simulink model "detumbling_group24"  (R2023b)
settings: Solver=ode4  StartTime=0.0  StopTime=stopTime  FixedStep=0.1  RelTol=1e-3
values from neighbouring files (symbols this model uses):
  a = 6939    [Air_Drag_script.m]    (also in main.m = 6939.063; main_group24.m = 6939.063)
  A0 = eye(3)    [Air_Drag_script.m]    (also in main_group24.m)
  ARW = 0.15    [main_group24.m]
  by = 0.1    [main_group24.m]
  bz = 0.1    [main_group24.m]
  c = 2.99792*10^8    (= 299792000)    [main.m]    (also in main_group24.m)
  e = 0    [Air_Drag_script.m]    (also in main.m = 0.001304; main_group24.m = 0.001304)
  G = [gn, gm, gvali, gsvi]    [main.m]    (also in main_group24.m)
  GyroSampleRate = 10    [main_group24.m]
  H = [hn, hm, hvali, hsvi]    [main.m]    (also in main_group24.m)
  i = deg2rad(97.5307)    [Air_Drag_script.m]    (also in main.m; main_group24.m)
  inertia1 = Iz-Iy    (= -0.016811111)    [main.m]    (also in main_group24.m = -0.0205003333333)
  inertia2 = Ix-Iz    (= 0.033125546)    [main.m]    (also in main_group24.m = 0.0205003333333)
  inertia3 = Iy-Ix    (= -0.016314435)    [main.m]    (also in main_group24.m = 0)
  Inertia_matrix = [Ix 0 0; 0 Iy 0; 0 0 Iz]    [main.m]
  Inverse_inertia = inv(Inertia_matrix)    [main.m]
  Ix = J(1,1)    [Air_Drag_script.m]    (also in data_mass.m = 0.0755003333333; main.m = 0.057749855; main_group24.m = 0.0755003333333)
  Iy = J(2,2)    [Air_Drag_script.m]    (also in data_mass.m = 0.0755003333333; main.m = 0.04143542; main_group24.m = 0.0755003333333)
  Iz = J(3,3)    [Air_Drag_script.m]    (also in data_mass.m = 0.055; main.m = 0.024624309; main_group24.m = 0.055)
  Ld = 1e-5    (= 1e-05)    [main_group24.m]
  Lw = 0.8    [main_group24.m]
  m = [0.1; 0.1; 0.1]    [main.m]    (also in main_group24.m)
  MB = [4; 0.1; 0.1; 0.3]    [main.m]    (also in main_group24.m)
  MMnoise = 15e-9*[1; 1; 1]    [main_group24.m]
  MMSampleRate = 1    [main_group24.m]
  mu = 3.98600433e+5    (= 398600.433)    [main.m]    (also in main_group24.m)
  n = 0.0011    [Air_Drag_script.m]    (also in main.m = sqrt(mu/a^3); main_group24.m = sqrt(mu/a^3))
  q0 = [ 1 1 1 1 ]'    [Air_Drag_script.m]    (also in main_group24.m = [0 0 0 1]')
  R_e = 6378    [main.m]    (also in main_group24.m)
  rho_d_MB = 0.1    [main.m]    (also in main_group24.m)
  rho_d_SP = 0.1    [main.m]    (also in main_group24.m)
  rho_s_MB = 0.5    [main.m]    (also in main_group24.m)
  rho_s_SP = 0.1    [main.m]    (also in main_group24.m)
  RRW = 0.3    [main_group24.m]
  SP = [1; 0.3; 0.1; 0.01]    [main.m]    (also in main_group24.m = [0.25; 0.1; 0.3; 0.01])
  w0 = [0 0 0]'    [Air_Drag_script.m]    (also in main.m = [wx0; wy0; wz0]; main_group24.m = [wx0; wy0; wz0])
undefined symbols (not defined in the file or in its folder): thrust
libraries: matrix_library x8, vrlib x2, simulink_extras x1, slpidlib x1, sharedutil x1
(part 1 of 3)
settings Model: Creator=hp  LastModifiedBy=hp

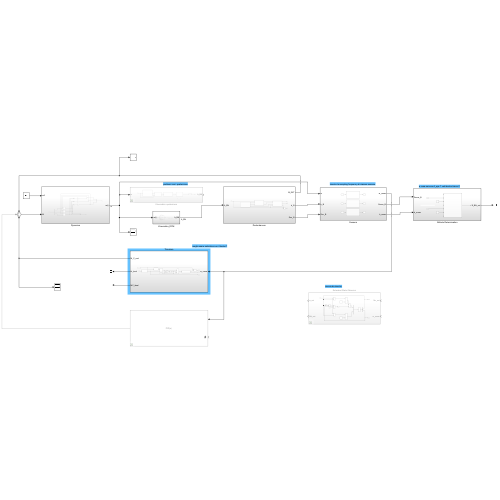
[thumbnail: Simulink's stored preview of the top-level diagram]
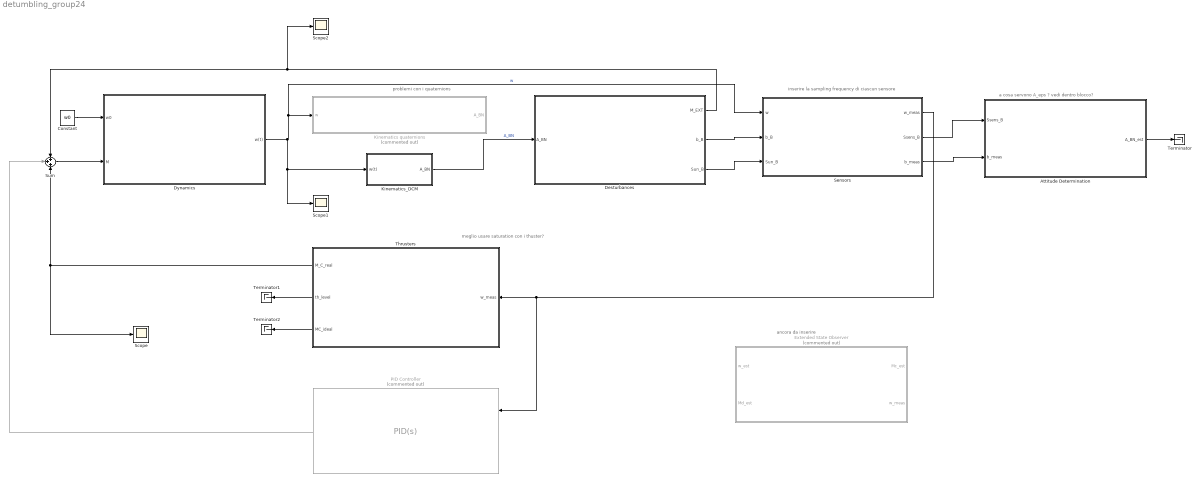
== system detumbling_group24 ==
  note: meglio usare saturation con i thuster?
  note: a cosa servono A_eps ? vedi dentro blocco?
  note: inserire la sampling frequency di ciascun sensore
  note: ancora da inserire
  note: problemi con i quaternions
  Attitude Determination : Subsystem
  Constant : Constant  Value=w0  VectorParams1D=off
  Desturbances : Subsystem
  Dynamics : Subsystem
  Extended State Observer : Subsystem  Commented=on
  Kinematics quaternions : Subsystem  Commented=on
  Kinematics_DCM : Subsystem
  PID Controller : slpidlib/PID Controller  Commented=on  Controller=PID  Form=Parallel  TimeDomain=Continuous-time  UseExternalTs=off  SampleTime=-1  IntegratorMethod=Forward Euler  FilterMethod=Forward Euler  ControllerParametersSource=internal  P=1000  I=0.1  UseKiTs=off  D=20  N=100  UseFilter=on  TunerSelectOption=Transfer Function Based (PID Tuner App)  InitialConditionSource=internal  InitialConditionForIntegrator=0  InitialConditionForFilter=0  DifferentiatorICPrevScaledInput=0  ExternalReset=level  TrackingMode=off  Kt=1  LimitOutput=off  SatLimitsSource=internal  UpperSaturationLimit=inf  LowerSaturationLimit=-inf  LinearizeAsGain=on  AntiWindupMode=none  Kb=1  LimitIntegrator=off  UpperIntegratorSaturationLimit=inf  LowerIntegratorSaturationLimit=-inf  POutMin=[]  POutMax=[]  IOutMin=[]  IOutMax=[]  DOutMin=[]  DOutMax=[]  NOutMin=[]  NOutMax=[]  SumOutMin=[]  SumOutMax=[]  SaturationOutMin=[]  SaturationOutMax=[]  PParamMin=[]  PParamMax=[]  IParamMin=[]  IParamMax=[]  DParamMin=[]  DParamMax=[]  NParamMin=[]  NParamMax=[]  KbParamMin=[]  KbParamMax=[]  KtParamMin=[]  KtParamMax=[]  KbOutMin=[]  KbOutMax=[]  KtOutMin=[]  KtOutMax=[]  IntegratorOutMin=[]  IntegratorOutMax=[]  FilterOutMin=[]  FilterOutMax=[]  SumI1OutMin=[]  SumI1OutMax=[]  SumI2OutMin=[]  SumI2OutMax=[]  SumI3OutMin=[]  SumI3OutMax=[]  SumI4OutMin=[]  SumI4OutMax=[]  SumDOutMin=[]  SumDOutMax=[]  DifferentiatorOutMin=[]  DifferentiatorOutMax=[]  FilterDiffOutCoefMin=[]  FilterDiffOutCoefMax=[]  ReciprocalOutMin=[]  ReciprocalOutMax=[]  SumDenOutMin=[]  SumDenOutMax=[]  SumNumOutMin=[]  SumNumOutMax=[]  DivideOutMin=[]  DivideOutMax=[]  UdiffTsProdOutMin=[]  UdiffTsProdOutMax=[]  NTsProdOutMin=[]  NTsProdOutMax=[]  UintegralTsProdOutMin=[]  UintegralTsProdOutMax=[]  UngainTsProdOutMin=[]  UngainTsProdOutMax=[]  ClampingZeroOutDataTypeStr=Inherit: Inherit via back propagation  ClampingZeroOutMin=[]  ClampingZeroOutMax=[]  FilterDenConstantOutDataTypeStr=Inherit: Inherit via back propagation  FilterDenConstantOutMin=[]  FilterDenConstantOutMax=[]  PCopyOutDataTypeStr=Inherit: Inherit via back propagation  PCopyOutMin=[]  PCopyOutMax=[]  NCopyOutDataTypeStr=Inherit: Inherit via back propagation  NCopyOutMin=[]  NCopyOutMax=[]  IntegratorContinuousStateAttributes=''  IntegratorStateMustResolveToSignalObject=off  IntegratorRTWStateStorageClass=Auto  FilterContinuousStateAttributes=''  FilterStateMustResolveToSignalObject=off  FilterRTWStateStorageClass=Auto  ParallelPVariant=InternalParameters  IdealPVariant=Disabled  IVariant=InternalParameters  DVariant=InternalParameters  IntegratorVariant=Continuous  SatVariant=Disabled  AWVariant=Passthrough  PCopyVariant=Disabled  TRVariant=Disabled  FdbkBlocksVariant=Forward  IdealPFdbkVariant=Disabled  SatFdbkVariant=Disabled  DerivativeFilterVariant=ContFilter  NVariant=InternalParameters  NCopyVariant=Disabled  FilterICVariant=InternalICsFilter  IntegratorICVariant=InternalICs  ExternalResetVariant=ExternalReset  TRSumVariant=Passthrough  SumFdbkVariant=Disabled  SumVariant=Sum_PID  TsampFilterVariant=InternalTs  TsampNgainVariant=Passthrough  TsampIntegralVariant=Disabled_SignalSpec  ExternalSaturationOutDataTypeStr=Inherit: Same as second input
  Scope : Scope
  Scope1 : Scope
  Scope2 : Scope
  Sensors : Subsystem
  Sum : Sum  Inputs=+++
  Terminator : Terminator
  Terminator1 : Terminator
  Terminator2 : Terminator
  Thrusters : Subsystem
  wires:
  Sensors/3(b_meas) -> Attitude Determination/2(b_meas)
  Sensors/2(Ssens_B) -> Attitude Determination/1(Ssens_B)
  Dynamics/1(w(t)) -> Scope1/1, Kinematics_DCM/1(w(t)), Sensors/1(w), Kinematics quaternions/1(w)  "w"
  Desturbances/2(b_B) -> Sensors/2(b_B)
  Sensors/1(w_meas) -> PID Controller/1, Thrusters/1(w_meas)
  Desturbances/3(Sun_B) -> Sensors/3(Sun_B)
  Sum/1 -> Dynamics/2(M)
  Thrusters/1(M_C_real) -> Sum/3, Scope/1
  Desturbances/1(M_EXT) -> Scope2/1, Sum/1
  Attitude Determination/1(A_BN_est) -> Terminator/1
  Thrusters/3(MC_ideal) -> Terminator2/1
  Thrusters/2(th_level) -> Terminator1/1
  Constant/1 -> Dynamics/1(w0)
  Kinematics_DCM/1(A_BN) -> Desturbances/1(A_BN)  "A_BN"
  PID Controller/1 -> Sum/2

== system detumbling_group24/Attitude Determination ==
  note: perchè aggiungere ancora A_eps?????
  Ssens_B : Inport
  b_meas : Inport  Port=2
  Attitude Determination : MATLAB Function  TreatAsAtomicUnit=on
  Constant : Constant
  Constant1 : Constant
  A_BN_est : Outport
  wires:
  Attitude Determination/1(A_BN_est) -> A_BN_est/1  "A_BN_est"
  b_meas/1 -> Attitude Determination/2(b_N)
  Ssens_B/1 -> Attitude Determination/5(r_N)
  Constant1/1 -> Attitude Determination/6(accuracy2)
  Constant/1 -> Attitude Determination/3(accuracy1)

== system detumbling_group24/Desturbances ==
  A_BN : Inport
  External Torques : Subsystem
  MatrixMultiply : Product  Multiplication=Matrix(*)
  Orbital Mechanics : Subsystem
  Relative Attitude : Subsystem
  M_EXT : Outport
  b_B : Outport  Port=2
  Sun_B : Outport  Port=3
  wires:
  Relative Attitude/1(A_BL.) -> External Torques/1(A_BL)
  Relative Attitude/2(r_L) -> External Torques/2(r_L)
  A_BN/1 -> External Torques/4(A_BN), MatrixMultiply/1, Relative Attitude/1(A_BN_ideal)
  Orbital Mechanics/1(theta) -> Relative Attitude/2(theta)
  Orbital Mechanics/2(r_N) -> Relative Attitude/3(r_N)
  Orbital Mechanics/3(r) -> External Torques/3(r)
  External Torques/1(M_EXT) -> M_EXT/1
  External Torques/2(b_B) -> b_B/1
  External Torques/3(Sun_N) -> MatrixMultiply/2
  MatrixMultiply/1 -> Sun_B/1

== system detumbling_group24/Dynamics ==
  w0 : Inport
  M : Inport  Port=2
  Demux : Demux  Outputs=3
  Demux1 : Demux  Outputs=3
  Gain : Gain  Gain=(Iy-Iz)/Ix
  Gain1 : Gain  Gain=(Iz-Ix)/Iy
  Gain2 : Gain  Gain=(Ix-Iy)/Iz
  Sum : Sum  Inputs=|++
  Sum1 : Sum  Inputs=|++
  Sum2 : Sum  Inputs=|++
  Vector Concatenate : Concatenate  NumInputs=3  Mode=Multidimensional array
  XZ : Product
  YX : Product
  ZY : Product
  wx : Integrator  InitialConditionSource=external
  wy : Integrator  InitialConditionSource=external
  wz : Integrator  InitialConditionSource=external
  w(t) : Outport
  wires:
  XZ/1 -> Gain1/1
  Demux/2 -> wy/2  "wy0"
  wx/1 -> XZ/1, Vector Concatenate/1, YX/1
  w0/1 -> Demux/1
  wy/1 -> Vector Concatenate/2, YX/2, ZY/2
  Demux/1 -> wx/2  "wx0"
  wz/1 -> ZY/1, Vector Concatenate/3, XZ/2
  YX/1 -> Gain2/1
  Demux/3 -> wz/2  "wz0"
  ZY/1 -> Gain/1
  Vector Concatenate/1 -> w(t)/1
  Gain2/1 -> Sum2/1
  Gain1/1 -> Sum1/1
  Gain/1 -> Sum/1
  Sum/1 -> wx/1
  Sum1/1 -> wy/1
  Sum2/1 -> wz/1
  Demux1/1 -> Sum/2  "Mx"
  Demux1/2 -> Sum1/2  "My"
  Demux1/3 -> Sum2/2  "Mz"
  M/1 -> Demux1/1

== system detumbling_group24/Extended State Observer ==
  Mc_est : Inport
  w_meas : Inport  Port=2
  Constant4 : Constant  Value=Lw
  Constant5 : Constant  Value=Ld
  Cross Product : vrlib/Utilities/Cross Product
  Demux1 : Demux  Outputs=2
  Gain : Gain  Gain=Inertia_matrix  Multiplication=Matrix(K*u)
  Gain1 : Gain  Gain=Inverse_inertia  Multiplication=Matrix(K*u)
  Integrator : Integrator  InitialCondition=[w0; [0; 0; 0]]
  Mux : Mux  Inputs=2
  Product4 : Product
  Product5 : Product
  Sum4 : Sum  Inputs=+-
  Sum5 : Sum  Inputs=+-
  Sum6 : Sum
  Sum7 : Sum  Inputs=+++
  w_est : Outport
  Md_est : Outport  Port=2
  wires:
  Gain/1 -> Cross Product/1
  Sum5/1 -> Product5/1
  Constant5/1 -> Product5/2
  Cross Product/1 -> Sum7/1
  Product5/1 -> Mux/2
  Demux1/1 -> Sum5/2, Cross Product/2, Gain/1, Sum4/2, w_est/1
  Sum7/1 -> Gain1/1
  Gain1/1 -> Sum6/2
  Product4/1 -> Sum6/1
  Sum6/1 -> Mux/1
  Demux1/2 -> Md_est/1, Sum7/2
  Mux/1 -> Integrator/1
  Mc_est/1 -> Sum7/3
  w_meas/1 -> Sum5/1, Sum4/1
  Integrator/1 -> Demux1/1
  Constant4/1 -> Product4/2
  Sum4/1 -> Product4/1

== system detumbling_group24/Kinematics quaternions ==
  w : Inport
  A_matrix : Subsystem
  Create Omega Matrix : Subsystem
  Kinematics_quaternions : Subsystem
  Normalizer : Subsystem
  Subsystem : Subsystem  Commented=on
  w_at_matrix : Subsystem
  A_BN : Outport
  wires:
  Kinematics_quaternions/1(q_vect) -> A_matrix/1(q_vect)
  A_matrix/1(A_BN) -> Normalizer/1(A_BN)
  w/1 -> Create Omega Matrix/2(w), w_at_matrix/1(w(t))
  Create Omega Matrix/1(Omega) -> Kinematics_quaternions/1(Omega)  "Omega"
  w_at_matrix/1("[-w^]") -> Create Omega Matrix/1("[w^]")  "[-w^]"
  Normalizer/1(Out1) -> A_BN/1

== system detumbling_group24/Kinematics_DCM ==
  w(t) : Inport
  Constant : Constant  Value=0
  Constant1 : Constant  Value=0
  Constant2 : Constant  Value=0
  Demux : Demux  Outputs=3
  Integrator : Integrator  InitialCondition=A0
  Matrix Concatenate : Concatenate  NumInputs=3  Mode=Multidimensional array
  MatrixMultiply : Product  Multiplication=Matrix(*)
  Multiply{,1..3} (4 alike) : Gain  Gain=-1
  Mux : Mux  Inputs=3
  Mux1 : Mux  Inputs=3
  Mux2 : Mux  Inputs=3
  Reshape : Reshape  OutputDimensionality=Row vector (2-D)
  Reshape1 : Reshape  OutputDimensionality=Row vector (2-D)
  Reshape2 : Reshape  OutputDimensionality=Row vector (2-D)
  Scope : Scope
  Subsystem : Subsystem
  A_BN : Outport
  wires:
  w(t)/1 -> Demux/1  "omega"
  MatrixMultiply/1 -> Integrator/1  "dA_dt"
  Matrix Concatenate/1 -> Multiply3/1  "omega_hat"
  Constant/1 -> Mux/1
  Demux/3 -> Mux1/1, Multiply/1  "w_z"
  Multiply/1 -> Mux/2
  Demux/2 -> Mux/3, Multiply2/1  "w_y"
  Constant1/1 -> Mux1/2
  Demux/1 -> Mux2/2, Multiply1/1  "w_x"
  Multiply1/1 -> Mux1/3
  Constant2/1 -> Mux2/3
  Multiply2/1 -> Mux2/1
  Mux/1 -> Reshape/1
  Mux1/1 -> Reshape1/1
  Mux2/1 -> Reshape2/1
  Multiply3/1 -> MatrixMultiply/1
  Reshape/1 -> Matrix Concatenate/1
  Reshape1/1 -> Matrix Concatenate/2
  Reshape2/1 -> Matrix Concatenate/3
  Integrator/1 -> Subsystem/1(In1), MatrixMultiply/2  "A_BN"
  Subsystem/1(Out2) -> Scope/1, A_BN/1

== system detumbling_group24/Sensors ==
  w : Inport
  b_B : Inport  Port=2
  Sun_B : Inport  Port=3
  Gyroscope : Subsystem
  Magnetometer : Subsystem
  Sun Sensor : Subsystem
  w_meas : Outport
  Ssens_B : Outport  Port=2
  b_meas : Outport  Port=3
  wires:
  w/1 -> Gyroscope/1(w)
  Gyroscope/1(w_meas) -> w_meas/1
  Sun Sensor/1(Ssens_B) -> Ssens_B/1
  Sun_B/1 -> Sun Sensor/1(Sun_B)
  b_B/1 -> Magnetometer/1(b_B)
  Magnetometer/1(MM_meas) -> b_meas/1

== system detumbling_group24/Thrusters ==
  w_meas : Inport
  Constant : Constant  Value=thrust.w
  Constant1 : Constant  Value=thrust.R
  Divide : Product  Inputs=*/
  Ideal control (detumbling) : Subsystem
  MATLAB Function : MATLAB Function  TreatAsAtomicUnit=on
  MATLAB Function1 : MATLAB Function  TreatAsAtomicUnit=on
  Matrix Multiply : Product  Multiplication=Matrix(*)
  Matrix Multiply1 : Product  Multiplication=Matrix(*)
  Max of Elements : MinMax  Function=max
  Product : Product
  Sum : Sum
  M_C_real : Outport
  th_level : Outport  Port=2
  MC_ideal : Outport  Port=3
  wires:
  Constant/1 -> Divide/2, Product/2  "w"
  Product/1 -> Sum/2
  Divide/1 -> Max of Elements/1
  Max of Elements/1 -> Product/1  "gamma"
  Ideal control (detumbling)/1(MC_ideal) -> MC_ideal/1, Matrix Multiply/2
  MATLAB Function1/1(y) -> Matrix Multiply/1
  Matrix Multiply1/1 -> M_C_real/1
  Sum/1 -> MATLAB Function/1(u_c)  "deal"
  Matrix Multiply/1 -> Divide/1, Sum/1
  MATLAB Function/1(u_c_real) -> Matrix Multiply1/2  "real"
  MATLAB Function/2(th_level) -> th_level/1
  w_meas/1 -> Ideal control (detumbling)/1(w)
  Constant1/1 -> Matrix Multiply1/1, MATLAB Function1/1(u)

== system detumbling_group24/Desturbances/External Torques ==
  A_BL : Inport
  r_L : Inport  Port=2
  r : Inport  Port=3
  A_BN : Inport  Port=4
  Constant : Constant  Value=MB
  Constant1 : Constant  Value=SP
  M_GG : Subsystem
  Magnetic field : Subsystem
  Solar radiation : Subsystem
  Sum of Elements : Sum  Inputs=+++
  To Workspace : ToWorkspace  VariableName=M_GG  SaveFormat=Timeseries  SampleTime=-1
  To Workspace1 : ToWorkspace  VariableName=M_SRP  SaveFormat=Timeseries  SampleTime=-1
  To Workspace2 : ToWorkspace  VariableName=M_MAG  SaveFormat=Timeseries  SampleTime=-1
  M_EXT : Outport
  b_B : Outport  Port=2
  Sun_N : Outport  Port=3
  wires:
  r/1 -> M_GG/2(r)
  Constant/1 -> Solar radiation/2(MB)
  Constant1/1 -> Solar radiation/3(SP)
  A_BN/1 -> Solar radiation/1(A_BN), Magnetic field/2(A_BN)
  Magnetic field/1(M_MAG) -> To Workspace2/1, Sum of Elements/3
  Sum of Elements/1 -> M_EXT/1
  A_BL/1 -> M_GG/1(A_BL)
  r_L/1 -> Magnetic field/1(r_L)
  M_GG/1(M_GG1) -> Sum of Elements/1, To Workspace/1
  Solar radiation/1(T_SRP) -> To Workspace1/1, Sum of Elements/2
  Magnetic field/2(b_B) -> b_B/1
  Solar radiation/2(Sun_N) -> Sun_N/1

== system detumbling_group24/Desturbances/Orbital Mechanics ==
  Sat Position magnitude : Subsystem
  Sat True Anomaly : Subsystem
  Sat position vector in inertial frame : Subsystem
  theta : Outport
  r_N : Outport  Port=2
  r : Outport  Port=3
  wires:
  Sat True Anomaly/1(theta) -> Sat position vector in inertial frame/2(theta), theta/1, Sat Position magnitude/1(theta)  "theta"
  Sat Position magnitude/1(r) -> r/1, Sat position vector in inertial frame/1(r)
  Sat position vector in inertial frame/1(r_N) -> r_N/1  "r_N"

== system detumbling_group24/Desturbances/Relative Attitude ==
  A_BN_ideal : Inport
  theta : Inport  Port=2
  r_N : Inport  Port=3
  A_BL : Subsystem
  A_LN : Subsystem
  MatrixMultiply : Product  Multiplication=Matrix(*)
  A_BL. : Outport
  r_L : Outport  Port=2
  wires:
  A_LN/1(A_LN) -> MatrixMultiply/1, A_BL/2(A_LN)
  theta/1 -> A_LN/1(theta)
  A_BN_ideal/1 -> A_BL/1(A_BN)
  A_BL/1(A_BL) -> A_BL./1
  r_N/1 -> MatrixMultiply/2
  MatrixMultiply/1 -> r_L/1

== system detumbling_group24/Kinematics quaternions/A_matrix ==
  q_vect : Inport
  Add : Sum  Inputs=++-
  Constant : Constant  Value=0
  Constant1 : Constant  Value=0
  Constant2 : Constant  Value=0
  Demux : Demux
  I : Constant  Value=eye(3)
  Matrix Concatenate : Concatenate  NumInputs=3  Mode=Multidimensional array
  MatrixMultiply : Product  Multiplication=Matrix(*)
  MatrixMultiply1 : Product
  MatrixMultiply2 : Product  Multiplication=Matrix(*)
  MatrixMultiply3 : Product
  Multiply : Gain  Gain=-1
  Multiply1 : Gain  Gain=-1
  Multiply2 : Gain  Gain=-1
  Multiply3 : Gain  Gain=2
  Multiply4 : Gain  Gain=2
  Mux{,1..3} (4 alike) : Mux  Inputs=3
  Reshape : Reshape  OutputDimensionality=Row vector (2-D)
  Reshape1 : Reshape  OutputDimensionality=Row vector (2-D)
  Reshape2 : Reshape  OutputDimensionality=Row vector (2-D)
  Square : Math  Operator=square
  Subtract : Sum  Inputs=-+
  Transpose : Math  Operator=transpose
  A_BN : Outport
  wires:
  q_vect/1 -> Demux/1
  Demux/1 -> Mux3/1, Mux2/2, Multiply1/1  "q1"
  Demux/2 -> Mux3/2, Mux/3, Multiply2/1  "q2"
  Demux/3 -> Mux3/3, Multiply/1, Mux1/1  "q3"
  Demux/4 -> Square/1, Multiply4/1  "q4"
  Mux/1 -> Reshape/1
  Reshape/1 -> Matrix Concatenate/1
  Mux1/1 -> Reshape1/1
  Mux2/1 -> Reshape2/1
  Reshape1/1 -> Matrix Concatenate/2
  Reshape2/1 -> Matrix Concatenate/3
  Multiply/1 -> Mux/2
  Constant1/1 -> Mux1/2
  Multiply1/1 -> Mux1/3
  Multiply2/1 -> Mux2/1
  Constant2/1 -> Mux2/3
  Matrix Concatenate/1 -> MatrixMultiply3/2  "q_hat"
  Mux3/1 -> MatrixMultiply2/1, Transpose/1, MatrixMultiply/2  "q_bar"
  Transpose/1 -> MatrixMultiply2/2, MatrixMultiply/1
  Square/1 -> Subtract/2
  MatrixMultiply/1 -> Subtract/1
  Subtract/1 -> MatrixMultiply1/1
  I/1 -> MatrixMultiply1/2
  MatrixMultiply2/1 -> Multiply3/1
  Multiply4/1 -> MatrixMultiply3/1
  Multiply3/1 -> Add/1
  MatrixMultiply1/1 -> Add/2
  MatrixMultiply3/1 -> Add/3
  Add/1 -> A_BN/1
  Constant/1 -> Mux/1

== system detumbling_group24/Kinematics quaternions/Create Omega Matrix ==
  "[w^]" : Inport
  w : Inport  Port=2
  " Col added" : Concatenate  Mode=Multidimensional array  ConcatenateDimension=2
  " Row added" : Concatenate  Mode=Multidimensional array
  Constant : Constant  Value=0
  Gain : Gain  Gain=-1
  Transpose : Math  Operator=transpose
  Vector Concatenate : Concatenate
  Omega : Outport
  wires:
  w/1 -> Transpose/1, Vector Concatenate/1
  Constant/1 -> Vector Concatenate/2
  Transpose/1 -> Gain/1
  "[w^]"/1 -> " Row added"/1
  " Row added"/1 -> " Col added"/1
  Vector Concatenate/1 -> " Col added"/2
  Gain/1 -> " Row added"/2
  " Col added"/1 -> Omega/1

== system detumbling_group24/Kinematics quaternions/Kinematics_quaternions ==
  Omega : Inport
  Constant : Constant  Value=q0  VectorParams1D=off
  Gain : Gain  Gain=0.5
  Integrator : Integrator  InitialConditionSource=external  InitialCondition=q0
  Omega*q(t) : Product  Multiplication=Matrix(*)
  Scope : Scope
  q_vect : Outport
  wires:
  Gain/1 -> Scope/1, q_vect/1, Integrator/1
  Integrator/1 -> Omega*q(t)/2  "q(t)"
  Omega*q(t)/1 -> Gain/1
  Omega/1 -> Omega*q(t)/1
  Constant/1 -> Integrator/2

== system detumbling_group24/Kinematics quaternions/Normalizer ==
  A_BN : Inport
  Gain : Gain  Gain=1.5
  Gain1 : Gain  Gain=0.5
  MatrixMultiply : Product  Multiplication=Matrix(*)
  MatrixMultiply1 : Product  Multiplication=Matrix(*)
  Sum : Sum  Inputs=+-
  Transpose : matrix_library/Transpose
  Out1 : Outport
  wires:
  A_BN/1 -> Transpose/1, MatrixMultiply/1, Gain/1, MatrixMultiply1/2
  Gain/1 -> Sum/1
  Sum/1 -> Out1/1
  Transpose/1 -> MatrixMultiply/2
  MatrixMultiply/1 -> MatrixMultiply1/1
  MatrixMultiply1/1 -> Gain1/1
  Gain1/1 -> Sum/2

== system detumbling_group24/Kinematics quaternions/Subsystem ==
  q_vect : Inport
  Demux : Demux
  From{,1..5} (6 alike) : From
  Goto{,1..8} (9 alike) : Goto
  Square{,1..3} (4 alike) : Math  Operator=square
  q1 q2 : Product
  q1 q3 : Product
  q1 q4 : Product
  q2 q4 : Product
  q3 q4 : Product
  Out1 : Outport
  wires:
  q_vect/1 -> Demux/1
  Demux/1 -> q1 q4/1, Square/1, q1 q3/1, q1 q2/1  "q1"
  Demux/2 -> Square1/1, q1 q2/2  "q2"
  Demux/3 -> q3 q4/2, Square2/1, q1 q3/2  "q3"
  Demux/4 -> q1 q4/2, q3 q4/1, Square3/1  "q4"
  q1 q2/1 -> Goto/1
  q1 q3/1 -> Goto1/1
  Square/1 -> Goto2/1
  Square1/1 -> Goto3/1
  Square2/1 -> Goto4/1
  Square3/1 -> Goto5/1
  q3 q4/1 -> Goto6/1
  q2 q4/1 -> Goto7/1
  q1 q4/1 -> Goto8/1

== system detumbling_group24/Kinematics quaternions/w_at_matrix ==
  w(t) : Inport
  Constant : Constant  Value=0  VectorParams1D=off
  Constant1 : Constant  Value=0
  Constant2 : Constant  Value=0
  Demux : Demux  Outputs=3
  Gain3 : Gain  Gain=-1
  Gain4 : Gain  Gain=-1
  Gain5 : Gain  Gain=-1
  Matrix Concatenate1 : Concatenate  NumInputs=3  Mode=Multidimensional array  ConcatenateDimension=2
  Mux1 : Mux  Inputs=3
  Mux2 : Mux  Inputs=3
  Mux3 : Mux  Inputs=3
  "[-w^]" : Outport
  wires:
  Demux/2 -> Mux1/3, Gain5/1  "wy"
  Gain3/1 -> Mux1/2
  Matrix Concatenate1/1 -> "[-w^]"/1
  Constant2/1 -> Mux3/3
  Demux/3 -> Mux2/1, Gain3/1  "wz"
  Constant1/1 -> Mux2/2
  Demux/1 -> Gain4/1, Mux3/2  "wx"
  Gain4/1 -> Mux2/3
  Mux1/1 -> Matrix Concatenate1/1
  Mux2/1 -> Matrix Concatenate1/2
  Gain5/1 -> Mux3/1
  Constant/1 -> Mux1/1
  Mux3/1 -> Matrix Concatenate1/3
  w(t)/1 -> Demux/1

== system detumbling_group24/Kinematics_DCM/Subsystem ==
  In1 : Inport
  Matrix Multiply : Product  Multiplication=Matrix(*)
  Matrix Multiply1 : Product  Multiplication=Matrix(*)
  Multiply : Gain  Gain=3/2
  Multiply1 : Gain  Gain=1/2
  Subtract : Sum  Inputs=+-
  Transpose : Math  Operator=transpose
  Out2 : Outport
  wires:
  Subtract/1 -> Out2/1
  Multiply1/1 -> Subtract/2
  Matrix Multiply1/1 -> Multiply1/1
  Multiply/1 -> Subtract/1
  Transpose/1 -> Matrix Multiply/2
  Matrix Multiply/1 -> Matrix Multiply1/1
  In1/1 -> Matrix Multiply1/2, Matrix Multiply/1, Multiply/1, Transpose/1  "A"

== system detumbling_group24/Sensors/Gyroscope ==
  note: w_BN_measured = G(w_B) A_eps w_BN + n + b
  w : Inport
  ARW : RandomNumber  Variance=(deg2rad(ARW)/sqrt(3600)/sqrt(1/GyroSampleRate))^2*[1;1;1]  SampleTime=1/GyroSampleRate
  Integrator : Integrator
  RRW : RandomNumber  Variance=(deg2rad(RRW)/3600/sqrt(1/GyroSampleRate))^2* [1;1;1]  SampleTime=1/GyroSampleRate
  Sum : Sum  Inputs=+++
  w_meas : Outport
  wires:
  RRW/1 -> Integrator/1  "b_dot"
  ARW/1 -> Sum/2  "n"
  Integrator/1 -> Sum/3  "b"
  Sum/1 -> w_meas/1
  w/1 -> Sum/1

== system detumbling_group24/Sensors/Magnetometer ==
  b_B : Inport
  Constant : Constant  Value=MMnoise
  MatrixMultiply : Product  Multiplication=Matrix(*)
  Subsystem : Subsystem
  Sum : Sum
  MM_meas : Outport
  wires:
  Constant/1 -> Sum/2
  b_B/1 -> Sum/1  "b_B"
  Subsystem/1(A_epsMM) -> MatrixMultiply/1
  Sum/1 -> MatrixMultiply/2
  MatrixMultiply/1 -> MM_meas/1

== system detumbling_group24/Sensors/Sun Sensor ==
  Sun_B : Inport
  Matrix Multiply1 : Product  Multiplication=Matrix(*)
  Subsystem : Subsystem
  Ssens_B : Outport
  wires:
  Sun_B/1 -> Matrix Multiply1/2
  Subsystem/1(A_eps) -> Matrix Multiply1/1  "A_eps"
  Matrix Multiply1/1 -> Ssens_B/1

== system detumbling_group24/Thrusters/Ideal control (detumbling) ==
  w : Inport
  Bracci thrusters : Constant  Value=[bz ; bz ; by]  VectorParams1D=off
  Gain3 : Gain  Gain=-1
  Matrix Multiply : Product
  Product2 : Product
  Sign : Signum
  variable T : MATLAB Function  TreatAsAtomicUnit=on
  MC_ideal : Outport
  wires:
  w/1 -> Sign/1, variable T/1(w)
  Matrix Multiply/1 -> Product2/1
  Product2/1 -> Gain3/1
  variable T/1(T) -> Matrix Multiply/2
  Bracci thrusters/1 -> Matrix Multiply/1
  Sign/1 -> Product2/2
  Gain3/1 -> MC_ideal/1

== system detumbling_group24/Desturbances/External Torques/M_GG ==
  A_BL : Inport
  r : Inport  Port=2
  GG Torque1 : Subsystem
  "c1, c2, c3" : Subsystem
  M_GG1 : Outport
  wires:
  "c1, c2, c3"/1(c1) -> GG Torque1/1(c1)
  "c1, c2, c3"/2(c2) -> GG Torque1/2(c2)
  "c1, c2, c3"/3(c3) -> GG Torque1/3(c3)
  A_BL/1 -> "c1, c2, c3"/1(A_BL)
  GG Torque1/1(M_GG) -> M_GG1/1
  r/1 -> GG Torque1/4(r)

== system detumbling_group24/Desturbances/External Torques/Magnetic field ==
  r_L : Inport
  A_BN : Inport  Port=2
  Clock : Clock
  Constant : Constant  Value=m
  Constant1 : Constant  Value=R_e*1000
  Constant3 : Constant  Value=G
  Constant4 : Constant  Value=H
  Cross Product1 : matrix_library/Cross Product
  MATLAB Function : MATLAB Function  TreatAsAtomicUnit=on
  MatrixMultiply : Product  Multiplication=Matrix(*)
  Reshape1 : Reshape  OutputDimensionality=Column vector (2-D)
  M_MAG : Outport
  b_B : Outport  Port=2
  wires:
  Constant1/1 -> MATLAB Function/2(r)
  Clock/1 -> MATLAB Function/3(t)
  Constant3/1 -> MATLAB Function/4(G)
  MATLAB Function/1(b_N) -> Reshape1/1
  r_L/1 -> MATLAB Function/1(r_LVLH)
  Reshape1/1 -> MatrixMultiply/2
  Constant4/1 -> MATLAB Function/5(H)
  A_BN/1 -> MatrixMultiply/1
  Constant/1 -> Cross Product1/1
  MatrixMultiply/1 -> b_B/1, Cross Product1/2
  Cross Product1/1 -> M_MAG/1

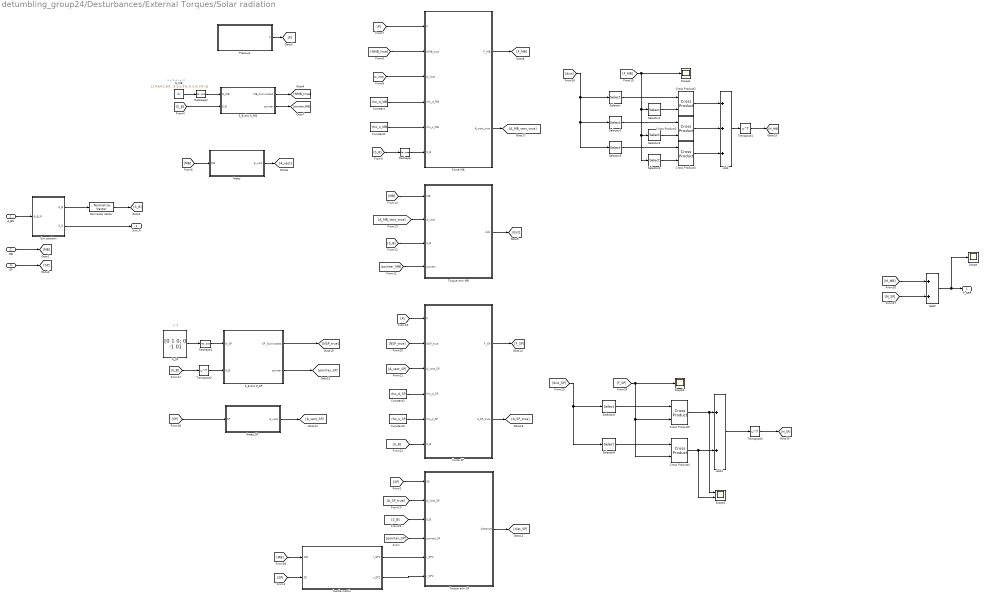
== system detumbling_group24/Desturbances/External Torques/Solar radiation ==
  note: x,y,z,-x,-y,-z
  note: y,-y
  A_BN : Inport
  MB : Inport  Port=2
  SP : Inport  Port=3
  Add : Sum  Inputs=3
  Add1 : Sum
  Add2 : Sum
  Areas : Subsystem
  Areas_SP : Subsystem
  Constant : Constant  Value=rho_d_MB
  Constant1 : Constant  Value=rho_s_MB
  Constant2 : Constant  Value=rho_d_SP
  Constant3 : Constant  Value=rho_s_SP
  Cross Product{1..5} (5 alike) : matrix_library/Cross Product
  Force MB : Subsystem
  Force SP : Subsystem
  Inertia matrix : Subsystem
  N_MB : Constant  Value=[1 0 0;0 1 0;0 0 1;-1 0 0; 0 -1 0; 0 0 -1]  VectorParams1D=off
  N_SP : Constant  Value=[0 1 0; 0 -1 0]  VectorParams1D=off
  Normalize Vector : vrlib/Utilities/Normalize Vector  maxzero=0
  Pressure : Subsystem
  Reshape : Reshape  OutputDimensionality=Column vector (2-D)
  Reshape1 : Reshape  OutputDimensionality=Customize  OutputDimensions=[2,3]
  Reshape2 : Reshape  OutputDimensionality=Customize  OutputDimensions=[6,3]
  S_B dot N_MB : Subsystem
  S_B dot N_SP : Subsystem
  Scope : Scope
  Scope1 : Scope
  Scope2 : Scope  NumInputPorts=2
  Scope3 : Scope
  Selector : Selector  NumberOfDimensions=2  InputPortWidth=3  IndexOptions=Index vector (dialog),Index vector (dialog)  Indices=1,[1 2 3]  OutputSizes=1,1
  Selector1 : Selector  NumberOfDimensions=2  InputPortWidth=3  IndexOptions=Index vector (dialog),Index vector (dialog)  Indices=1,[1 2 3]  OutputSizes=1,1
  Selector2 : Selector  NumberOfDimensions=2  InputPortWidth=3  IndexOptions=Index vector (dialog),Index vector (dialog)  Indices=2,[1 2 3]  OutputSizes=1,1
  Selector3 : Selector  NumberOfDimensions=2  InputPortWidth=3  IndexOptions=Index vector (dialog),Index vector (dialog)  Indices=2,[1 2 3]  OutputSizes=1,1
  Selector4 : Selector  NumberOfDimensions=2  InputPortWidth=3  IndexOptions=Index vector (dialog),Index vector (dialog)  Indices=3,[1 2 3]  OutputSizes=1,1
  Selector5 : Selector  NumberOfDimensions=2  InputPortWidth=3  IndexOptions=Index vector (dialog),Index vector (dialog)  Indices=3,[1 2 3]  OutputSizes=1,1
  Selector6 : Selector  NumberOfDimensions=2  InputPortWidth=3  IndexOptions=Index vector (dialog),Index vector (dialog)  Indices=1,[1 2 3]  OutputSizes=1,1
  Selector8 : Selector  NumberOfDimensions=2  InputPortWidth=3  IndexOptions=Index vector (dialog),Index vector (dialog)  Indices=2,[1 2 3]  OutputSizes=1,1
  Sun position : Subsystem
  Torque arm MB : Subsystem
  Torque arm SP : Subsystem
  Transpose1 : Math  Operator=transpose
  Transpose2 : Math  Operator=transpose
  Transpose3 : Math  Operator=transpose
  T_SRP : Outport
  Sun_N : Outport  Port=2
  wires:
  Sun position/1(S_B) -> Normalize Vector/1
  MB/1 -> [MB]
  N_MB/1 -> Reshape2/1
  [NMB_true] -> Force MB/2(NMB_true)
  S_B dot N_MB/1(MB_illuminated) -> [NMB_true]
  [MB] -> Areas/1(MB)
  [S_B] -> S_B dot N_MB/2(S_B)
  Sun position/2(S_N) -> Sun_N/1
  [P] -> Force MB/1(P)
  Areas/1(A_vect) -> [A_vect]
  Transpose1/1 -> [M_MB]
  Areas_SP/1(A_vect) -> [A_vect_SP]
  Reshape1/1 -> S_B dot N_SP/1(N_SP)
  Transpose3/1 -> [M_SP]
  Selector2/1 -> Cross Product1/1
  [MB] -> Torque arm MB/1(MB)
  Constant3/1 -> Force SP/5(rho_s_SP)
  [F_SP] -> Cross Product5/2, Cross Product4/2, Scope3/1
  [M_MB] -> Add2/1
  [dist_SP] -> Selector6/1, Selector8/1
  [pointer_SP] -> Torque arm SP/4(pointer_SP)
  Cross Product4/1 -> Scope2/2, Add1/2
  [F_MB] -> Scope1/1, Selector4/1, Selector3/1, Selector1/1
  A_BN/1 -> Sun position/1(A_B_N)
  Add1/1 -> Transpose3/1
  Transpose2/1 -> S_B dot N_SP/2(S_B)
  [SP] -> Areas_SP/1(SP)
  [A_SP_true] -> Torque arm SP/2(A_vect_SP)
  Add/1 -> Transpose1/1
  Torque arm SP/1(distance) -> [dist_SP]
  Reshape2/1 -> S_B dot N_MB/1(N_MB)
  Torque arm MB/1(dist) -> [dist]
  S_B dot N_SP/2(pointer) -> [pointer_SP]
  Force MB/1(F_MB) -> [F_MB]
  Selector/1 -> Cross Product2/1
  [S_B] -> Reshape/1
  [P] -> Force SP/1(P)
  [A_vect] -> Force MB/3(A_vect)
  Selector1/1 -> Cross Product2/2
  Constant1/1 -> Force MB/5(rho_s_MB)
  [A_MB_vect_true] -> Torque arm MB/2(A_vect)
  Pressure/1(P) -> [P]
  Normalize Vector/1 -> [S_B]
  Constant2/1 -> Force SP/4(rho_d_SP)
  Constant/1 -> Force MB/4(rho_d_MB)
  Selector8/1 -> Cross Product4/1
  [dist] -> Selector2/1, Selector5/1, Selector/1
  [NSP_true] -> Force SP/2(NSP_true)
  N_SP/1 -> Reshape1/1
  [S_B] -> Torque arm MB/3(S_B)
  Force SP/2(A_SP_true) -> [A_SP_true]
  [S_B] -> Torque arm SP/3(S_B)
  SP/1 -> [SP]
  Selector4/1 -> Cross Product3/2
  S_B dot N_MB/2(pointer) -> [pointer_MB]
  Force MB/2(A_vect_true) -> [A_MB_vect_true]
  [pointer_MB] -> Torque arm MB/4(pointer)
  Add2/1 -> Scope/1, T_SRP/1
  Selector3/1 -> Cross Product1/2
  [S_B] -> Force SP/6(S_B)
  [S_B] -> Transpose2/1
  Cross Product5/1 -> Scope2/1, Add1/1
  [A_vect_SP] -> Force SP/3(A_vect_SP)
  Reshape/1 -> Force MB/6(S_B)
  Cross Product2/1 -> Add/1
  Force SP/1(F_SP) -> [F_SP]
  S_B dot N_SP/1(SP_illuminated) -> [NSP_true]
  Selector6/1 -> Cross Product5/1
  Selector5/1 -> Cross Product3/1
  Cross Product1/1 -> Add/2
  [M_SP] -> Add2/2
  [SP] -> Torque arm SP/1(SP)
  Cross Product3/1 -> Add/3
  [SP] -> Inertia matrix/2(SP)
  [MB] -> Inertia matrix/1(MB)
  Inertia matrix/1(r_SP1) -> Torque arm SP/5(r_SP1)
  Inertia matrix/2(r_SP2) -> Torque arm SP/6(r_SP2)

== system detumbling_group24/Desturbances/Orbital Mechanics/Sat Position magnitude ==
  note: 1+e cos(theta)
  note: a(1-e^2)
  note: Denominator
  note: Numerator
  theta : Inport
  Constant : Constant  Value=a
  Constant1 : Constant
  Constant3 : Constant  Value=e
  Constant4 : Constant
  Constant5 : Constant  Value=e
  Cos : Trigonometry  Operator=cos
  Divide : Product  Inputs=*/
  Product : Product
  Product1 : Product
  Square1 : Math  Operator=square
  Sum : Sum
  Sum1 : Sum  Inputs=+-
  r : Outport
  wires:
  Product1/1 -> Sum/1
  Sum1/1 -> Product/2
  Constant1/1 -> Sum1/1
  Sum/1 -> Divide/2
  Square1/1 -> Sum1/2
  Constant3/1 -> Product1/2
  Constant4/1 -> Sum/2
  Constant/1 -> Product/1
  Constant5/1 -> Square1/1
  Cos/1 -> Product1/1
  Product/1 -> Divide/1
  theta/1 -> Cos/1
  Divide/1 -> r/1

== system detumbling_group24/Desturbances/Orbital Mechanics/Sat True Anomaly ==
  note: (1-e^2)^3/2
  note: n ( 1+e cos(theta))^2
  note: Denominator
  note: Numerator
  Constant : Constant  Value=n
  Constant1 : Constant
  Constant2 : Constant  Value=e
  Constant3 : Constant
  Constant4 : Constant  Value=e
  Constant5 : Constant  Value=3/2
  Cos : Trigonometry  Operator=cos
  Divide : Product  Inputs=*/
  Integrator : Integrator
  Power : Math  Operator=pow
  Product : Product
  Product1 : Product
  Square : Math  Operator=square
  Square1 : Math  Operator=square
  Sum : Sum
  Sum1 : Sum  Inputs=|+-
  theta : Outport
  wires:
  Sum/1 -> Square/1
  Integrator/1 -> theta/1, Cos/1  "theta"
  Square/1 -> Product1/2
  Constant5/1 -> Power/2
  Constant3/1 -> Sum1/1
  Product1/1 -> Divide/1
  Constant/1 -> Product1/1
  Divide/1 -> Integrator/1  "theta_dot"
  Square1/1 -> Sum1/2
  Product/1 -> Sum/2
  Power/1 -> Divide/2
  Constant1/1 -> Sum/1
  Constant2/1 -> Product/1
  Constant4/1 -> Square1/1
  Cos/1 -> Product/2
  Sum1/1 -> Power/1

== system detumbling_group24/Desturbances/Orbital Mechanics/Sat position vector in inertial frame ==
  note: r_N = r [cos(theta)
      | 		sin(theta)cos(i)
      | 		sin(theta)sin(i)]
  r : Inport
  theta : Inport  Port=2
  Cos : Trigonometry  Operator=cos
  Cos1 : Trigonometry  Operator=cos
  Orbit Inclination : Constant  Value=i
  Product : Product
  Product1 : Product
  Product2 : Product
  Sin : Trigonometry
  Sin1 : Trigonometry
  Vector Concatenate : Concatenate  NumInputs=3  Mode=Multidimensional array
  r_N : Outport
  wires:
  Sin/1 -> Product1/1, Product/1
  Product/1 -> Vector Concatenate/2
  Sin1/1 -> Product1/2
  r/1 -> Product2/1
  Orbit Inclination/1 -> Sin1/1, Cos1/1
  Vector Concatenate/1 -> Product2/2
  theta/1 -> Cos/1, Sin/1
  Cos/1 -> Vector Concatenate/1
  Cos1/1 -> Product/2
  Product1/1 -> Vector Concatenate/3
  Product2/1 -> r_N/1

== system detumbling_group24/Desturbances/Relative Attitude/A_BL ==
  A_BN : Inport
  A_LN : Inport  Port=2
  Matrix Multiply : Product  Multiplication=Matrix(*)
  To Workspace : ToWorkspace  VariableName=A_BL  SampleTime=-1
  Transpose1 : matrix_library/Transpose
  A_BL : Outport
  wires:
  A_BN/1 -> Matrix Multiply/1
  A_LN/1 -> Transpose1/1
  Transpose1/1 -> Matrix Multiply/2
  Matrix Multiply/1 -> A_BL/1, To Workspace/1

== system detumbling_group24/Desturbances/Relative Attitude/A_LN ==
  theta : Inport
  Constant : Constant  Value=0
  Constant1 : Constant  Value=[0; 0; 1]
  Constant2 : Constant  Value=[1 0 0; 0 cos(i) sin(i); 0 -sin(i) cos(i)]
  Cos : Trigonometry  Operator=cos
  Gain : Gain  Gain=[1; -1; 1]
  Matrix Concatenate : Concatenate  NumInputs=3  Mode=Multidimensional array  ConcatenateDimension=2
  Product : Product  Multiplication=Matrix(*)
  Selector : Selector  InputPortWidth=3  IndexOptions=Index vector (dialog)  Indices=[3 2 1]  OutputSizes=1
  Selector1 : Selector  InputPortWidth=3  IndexOptions=Index vector (dialog)  Indices=[2 3 1]  OutputSizes=1
  Sin : Trigonometry
  To Workspace : ToWorkspace  VariableName=A_LN  SampleTime=-1
  Vector Concatenate : Concatenate  NumInputs=3
  A_LN : Outport
  wires:
  Matrix Concatenate/1 -> Product/1
  theta/1 -> Sin/1, Cos/1
  Gain/1 -> Matrix Concatenate/1
  Vector Concatenate/1 -> Selector1/1, Selector/1
  Sin/1 -> Vector Concatenate/3
  Selector/1 -> Matrix Concatenate/2
  Selector1/1 -> Gain/1
  Product/1 -> A_LN/1, To Workspace/1
  Constant1/1 -> Matrix Concatenate/3
  Cos/1 -> Vector Concatenate/2
  Constant/1 -> Vector Concatenate/1
  Constant2/1 -> Product/2

== system detumbling_group24/Sensors/Magnetometer/Subsystem ==
  Constant : Constant
  Display : Display
  Gain : Gain  Gain=[1; -1; 1]
  Gain1 : Gain  Gain=[1; 1; -1]
  Gain2 : Gain  Gain=[-1; 1; 1]
  Matrix Concatenate : Concatenate  NumInputs=3  Mode=Multidimensional array  ConcatenateDimension=2
  Random Number : RandomNumber  Variance=deg2rad(0.1)^2  Seed=5  SampleTime=1/MMSampleRate
  Random Number1 : RandomNumber  Variance=deg2rad(0.1)^2  Seed=6  SampleTime=1/MMSampleRate
  Random Number2 : RandomNumber  Variance=deg2rad(0.1)^2  Seed=7  SampleTime=1/MMSampleRate
  Selector : Selector  InputPortWidth=4  IndexOptions=Index vector (dialog)  Indices=[1 4 3]  OutputSizes=1
  Selector1 : Selector  InputPortWidth=4  IndexOptions=Index vector (dialog)  Indices=[4 1 2]  OutputSizes=1
  Selector2 : Selector  InputPortWidth=4  IndexOptions=Index vector (dialog)  Indices=[3 2 1]  OutputSizes=1
  Vector Concatenate : Concatenate  NumInputs=4
  A_epsMM : Outport
  wires:
  Selector2/1 -> Gain2/1
  Selector/1 -> Gain/1
  Gain/1 -> Matrix Concatenate/1
  Random Number/1 -> Vector Concatenate/2
  Matrix Concatenate/1 -> Display/1, A_epsMM/1
  Selector1/1 -> Gain1/1
  Vector Concatenate/1 -> Selector2/1, Selector/1, Selector1/1
  Gain2/1 -> Matrix Concatenate/3
  Constant/1 -> Vector Concatenate/1
  Gain1/1 -> Matrix Concatenate/2
  Random Number2/1 -> Vector Concatenate/4
  Random Number1/1 -> Vector Concatenate/3

== system detumbling_group24/Sensors/Sun Sensor/Subsystem ==
  note: A31
  note: A33
  note: A32
  note: A23
  note: A22
  note: A21
  note: A13
  note: A12
  note: A11
  Cos : Trigonometry  Operator=cos
  Cos1 : Trigonometry  Operator=cos
  Cos2 : Trigonometry  Operator=cos
  Create 3x3 Matrix : sharedutil/Create 3x3 Matrix  aMode=aMode
  Gain1 : Gain  Gain=-1
  Gain3 : Gain  Gain=-1
  Gain4 : Gain
  Product{,1,3,5..6,8,10..11} (8 alike) : Product
  Product{2,4,7,9} (4 alike) : Product  Inputs=3
  Sin : Trigonometry
  Sin1 : Trigonometry
  Sin2 : Trigonometry
  Sum : Sum
  Sum1 : Sum  Inputs=-+
  Sum2 : Sum  Inputs=-+
  Sum3 : Sum
  phi : RandomNumber  Variance=(1/8*pi/180)^2  Seed=2  SampleTime=0.2
  psi : RandomNumber  Variance=(1/8*pi/180)^2  SampleTime=0.2
  th : RandomNumber  Variance=(1/8*pi/180)^2  Seed=1  SampleTime=0.2
  A_eps : Outport
  wires:
  psi/1 -> Cos/1, Sin/1
  th/1 -> Sin1/1, Cos1/1
  phi/1 -> Sin2/1, Cos2/1
  Product2/1 -> Sum/1
  Product1/1 -> Sum/2
  Product3/1 -> Sum1/2
  Product4/1 -> Sum1/1
  Product7/1 -> Sum2/1
  Product6/1 -> Sum2/2
  Product9/1 -> Sum3/1
  Product8/1 -> Sum3/2
  Gain4/1 -> Create 3x3 Matrix/7  "A31"
  Product/1 -> Create 3x3 Matrix/1  "A11"
  Sum/1 -> Create 3x3 Matrix/2  "A12"
  Sum1/1 -> Create 3x3 Matrix/3  "A13"
  Product5/1 -> Gain1/1
  Sum2/1 -> Create 3x3 Matrix/5  "A22"
  Sum3/1 -> Create 3x3 Matrix/6  "A23"
  Product10/1 -> Gain3/1
  Product11/1 -> Create 3x3 Matrix/9  "A33"
  Gain1/1 -> Create 3x3 Matrix/4  "A21"
  Gain3/1 -> Create 3x3 Matrix/8  "A32"
  Cos/1 -> Product8/1, Product6/1, Product4/1, Product2/1, Product/1  "cos(psi)"
  Cos1/1 -> Product/2, Product11/1, Product10/1, Product5/2  "cos(th)"
  Sin1/1 -> Gain4/1, Product9/2, Product7/2, Product2/2, Product4/2  "sin(th)"
  Sin2/1 -> Product7/3, Product3/2, Product2/3, Product8/2, Product10/2  "sin(phi)"
  Sin/1 -> Product3/1, Product5/1, Product7/1, Product9/1, Product1/1  "sin(psi)"
  Cos2/1 -> Product6/2, Product4/3, Product1/2, Product9/3, Product11/2  "cos(phi)"
  Create 3x3 Matrix/1 -> A_eps/1  "A_eps"

== system detumbling_group24/Desturbances/External Torques/M_GG/GG Torque1 ==
  c1 : Inport
  c2 : Inport  Port=2
  c3 : Inport  Port=3
  r : Inport  Port=4
  Constant : Constant  Value=3
  Divide : Product  Inputs=*/
  Divide1 : Product  Inputs=*/
  Divide2 : Product  Inputs=*/
  Gain4 : Gain  Gain=3*mu
  Gain5 : Gain  Gain=3*mu
  Gain7 : Gain  Gain=3*mu
  Ix-Iz : Gain  Gain=inertia2
  Iy-Ix : Gain  Gain=inertia3
  Iz-Iy : Gain  Gain=inertia1
  Mux : Mux  Inputs=3
  Pow : Math  Operator=pow  RndMeth=Zero
  Product3 : Product
  Product4 : Product
  Product5 : Product
  M_GG : Outport
  wires:
  Pow/1 -> Divide2/2, Divide1/2, Divide/2
  Iz-Iy/1 -> Mux/1
  c3/1 -> Product3/2, Product4/2
  Product3/1 -> Gain4/1
  Divide2/1 -> Iy-Ix/1
  Gain4/1 -> Divide/1
  Gain5/1 -> Divide1/1
  Divide/1 -> Iz-Iy/1
  Constant/1 -> Pow/2
  Divide1/1 -> Ix-Iz/1
  Product5/1 -> Gain7/1
  c1/1 -> Product5/1, Product4/1
  r/1 -> Pow/1
  Iy-Ix/1 -> Mux/3
  Ix-Iz/1 -> Mux/2
  Gain7/1 -> Divide2/1
  Product4/1 -> Gain5/1
  c2/1 -> Product3/1, Product5/2
  Mux/1 -> M_GG/1

== system detumbling_group24/Desturbances/External Torques/M_GG/c1, c2, c3 ==
  A_BL : Inport
  Constant1 : Constant  Value=[1; 0; 0]
  Demux : Demux  Outputs=3
  Product1 : Product  Multiplication=Matrix(*)
  c1 : Outport
  c2 : Outport  Port=2
  c3 : Outport  Port=3
  wires:
  Demux/2 -> c2/1
  Product1/1 -> Demux/1
  Demux/1 -> c1/1
  Demux/3 -> c3/1
  Constant1/1 -> Product1/2
  A_BL/1 -> Product1/1

== system detumbling_group24/Desturbances/External Torques/Solar radiation/Areas ==
  MB : Inport
  Demux : Demux
  Mux : Mux  Inputs=3
  Product1 : Product
  Product2 : Product
  Product4 : Product
  Reshape : Reshape  OutputDimensionality=Column vector (2-D)
  Terminator : Terminator
  A_vect : Outport
  wires:
  Product2/1 -> Mux/2  "a*h"
  Product4/1 -> Mux/1  "b*h"
  MB/1 -> Demux/1
  Product1/1 -> Mux/3  "a*b"
  Demux/1 -> Terminator/1
  Demux/2 -> [a]
  Demux/3 -> [b]
  Demux/4 -> [h]
  [b] -> Product4/1
  [h] -> Product4/2
  [h] -> Product2/2
  [b] -> Product1/2
  [a] -> Product2/1
  [a] -> Product1/1
  Mux/1 -> Reshape/1
  Reshape/1 -> A_vect/1

== system detumbling_group24/Desturbances/External Torques/Solar radiation/Areas_SP ==
  SP : Inport
  Demux : Demux
  Product1 : Product
  Terminator : Terminator
  Terminator1 : Terminator
  A_vect : Outport
  wires:
  [a] -> Product1/1
  [b] -> Product1/2
  Demux/4 -> Terminator1/1
  Demux/3 -> [b]
  Demux/2 -> [a]
  Demux/1 -> Terminator/1
  Product1/1 -> A_vect/1  "a*b"
  SP/1 -> Demux/1

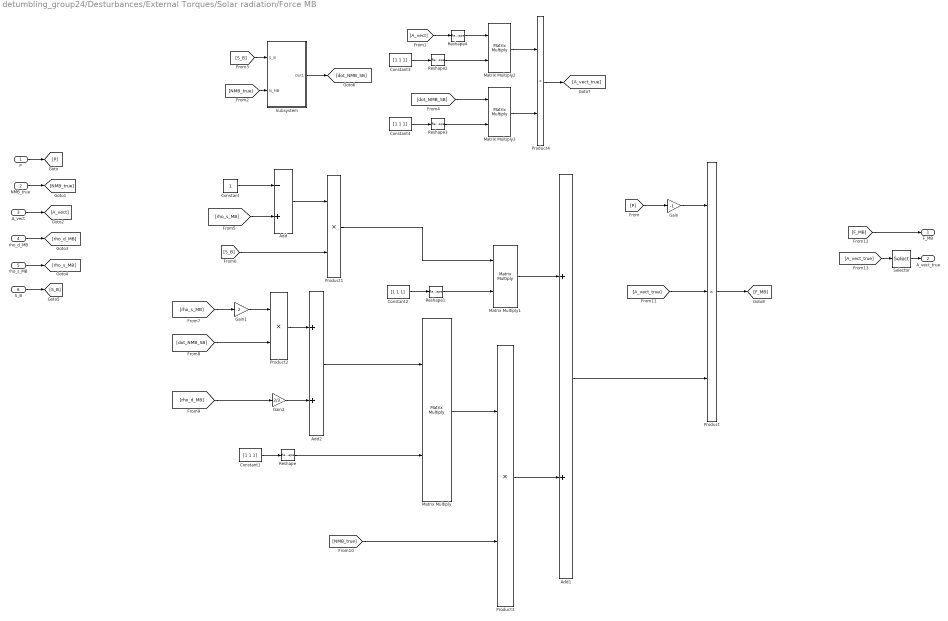
== system detumbling_group24/Desturbances/External Torques/Solar radiation/Force MB ==
  P : Inport
  NMB_true : Inport  Port=2
  A_vect : Inport  Port=3
  rho_d_MB : Inport  Port=4
  rho_s_MB : Inport  Port=5
  S_B : Inport  Port=6
  Add : Sum  Inputs=-+
  Add1 : Sum
  Add2 : Sum
  Constant : Constant
  Constant{1..4} (4 alike) : Constant  Value=[1 1 1]
  Gain : Gain  Gain=-1
  Gain1 : Gain  Gain=2
  Gain2 : Gain  Gain=2/3
  Matrix Multiply{,1..3} (4 alike) : Product  Multiplication=Matrix(*)
  Product : Product  Inputs=3
  Product{1..4} (4 alike) : Product
  Reshape{,1..3} (4 alike) : Reshape  OutputDimensionality=Row vector (2-D)
  Reshape4 : Reshape  OutputDimensionality=Column vector (2-D)
  Selector : Selector  NumberOfDimensions=2  InputPortWidth=3  IndexOptions=Index vector (dialog),Index vector (dialog)  Indices=[1 2 3],1  OutputSizes=1,1
  Subsystem : Subsystem
  F_MB : Outport
  A_vect_true : Outport  Port=2
  wires:
  P/1 -> [P]
  NMB_true/1 -> [NMB_true]
  A_vect/1 -> [A_vect]
  rho_d_MB/1 -> [rho_d_MB]
  rho_s_MB/1 -> [rho_s_MB]
  S_B/1 -> [S_B]
  [P] -> Gain/1
  Gain/1 -> Product/1
  [NMB_true] -> Subsystem/2(N_MB)
  [S_B] -> Subsystem/1(S_B)
  Subsystem/1(Out1) -> [dot_NMB_SB]
  [rho_s_MB] -> Add/2
  Constant/1 -> Add/1
  Add/1 -> Product1/1
  [S_B] -> Product1/2
  [rho_s_MB] -> Gain1/1
  [dot_NMB_SB] -> Product2/2
  Gain1/1 -> Product2/1
  Product2/1 -> Add2/1
  Gain2/1 -> Add2/2
  [rho_d_MB] -> Gain2/1
  [NMB_true] -> Product3/2
  Product3/1 -> Add1/2
  Add1/1 -> Product/3
  Constant1/1 -> Reshape/1
  Matrix Multiply/1 -> Product3/1
  Add2/1 -> Matrix Multiply/1
  Reshape/1 -> Matrix Multiply/2
  Matrix Multiply1/1 -> Add1/1
  Product1/1 -> Matrix Multiply1/1
  Constant2/1 -> Reshape1/1
  Reshape1/1 -> Matrix Multiply1/2
  Reshape2/1 -> Matrix Multiply2/2
  Constant3/1 -> Reshape2/1
  Reshape3/1 -> Matrix Multiply3/2
  Constant4/1 -> Reshape3/1
  [A_vect] -> Reshape4/1
  Reshape4/1 -> Matrix Multiply2/1
  [dot_NMB_SB] -> Matrix Multiply3/1
  Matrix Multiply2/1 -> Product4/1
  Matrix Multiply3/1 -> Product4/2
  Product4/1 -> [A_vect_true]
  [A_vect_true] -> Product/2
  Product/1 -> [F_MB]
  [F_MB] -> F_MB/1
  [A_vect_true] -> Selector/1
  Selector/1 -> A_vect_true/1

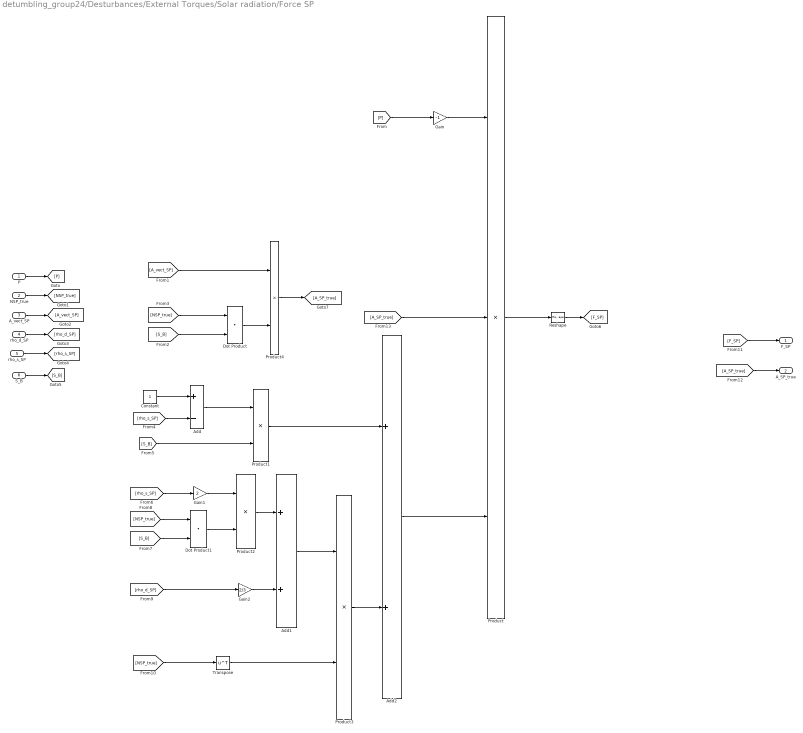
== system detumbling_group24/Desturbances/External Torques/Solar radiation/Force SP ==
  P : Inport
  NSP_true : Inport  Port=2
  A_vect_SP : Inport  Port=3
  rho_d_SP : Inport  Port=4
  rho_s_SP : Inport  Port=5
  S_B : Inport  Port=6
  Add : Sum  Inputs=+-
  Add1 : Sum
  Add2 : Sum
  Constant : Constant
  Dot Product : DotProduct  OutDataTypeStr=Inherit: Inherit via internal rule
  Dot Product1 : DotProduct  OutDataTypeStr=Inherit: Inherit via internal rule
  Gain : Gain  Gain=-1
  Gain1 : Gain  Gain=2
  Gain2 : Gain  Gain=2/3
  Product : Product  Inputs=3
  Product{1..4} (4 alike) : Product
  Reshape : Reshape  OutputDimensionality=Row vector (2-D)
  Transpose : Math  Operator=transpose
  F_SP : Outport
  A_SP_true : Outport  Port=2
  wires:
  P/1 -> [P]
  NSP_true/1 -> [NSP_true]
  A_vect_SP/1 -> [A_vect_SP]
  rho_d_SP/1 -> [rho_d_SP]
  rho_s_SP/1 -> [rho_s_SP]
  S_B/1 -> [S_B]
  Product/1 -> Reshape/1
  [P] -> Gain/1
  Gain/1 -> Product/1
  [S_B] -> Dot Product/2
  [NSP_true] -> Dot Product/1
  Constant/1 -> Add/1
  [rho_s_SP] -> Add/2
  Add/1 -> Product1/1
  [S_B] -> Product1/2
  [rho_s_SP] -> Gain1/1
  [NSP_true] -> Dot Product1/1
  [S_B] -> Dot Product1/2
  Dot Product1/1 -> Product2/2
  Gain1/1 -> Product2/1
  Product2/1 -> Add1/1
  [rho_d_SP] -> Gain2/1
  Gain2/1 -> Add1/2
  [NSP_true] -> Transpose/1
  Add1/1 -> Product3/1
  Product1/1 -> Add2/1
  Product3/1 -> Add2/2
  Transpose/1 -> Product3/2
  Add2/1 -> Product/3
  Reshape/1 -> [F_SP]
  [F_SP] -> F_SP/1
  Dot Product/1 -> Product4/2
  [A_vect_SP] -> Product4/1
  Product4/1 -> [A_SP_true]
  [A_SP_true] -> A_SP_true/1
  [A_SP_true] -> Product/2

== system detumbling_group24/Desturbances/External Torques/Solar radiation/Inertia matrix ==
  MB : Inport
  SP : Inport  Port=2
  Demux : Demux
  Demux1 : Demux
  Terminator{,1..5} (6 alike) : Terminator
  r_SP : Subsystem
  r_SP1 : Outport
  r_SP2 : Outport  Port=2
  wires:
  [a_MB] -> r_SP/2(a_MB)
  Demux/1 -> Terminator5/1
  SP/1 -> Demux/1
  Demux1/2 -> [a_MB]
  Demux1/3 -> Terminator/1
  Demux1/1 -> Terminator2/1
  Demux1/4 -> Terminator1/1
  MB/1 -> Demux1/1
  Demux/4 -> Terminator3/1
  Demux/2 -> Terminator4/1
  r_SP/2(r_SP2) -> r_SP2/1
  Demux/3 -> [b_SP]
  [b_SP] -> r_SP/1(b_SP)
  r_SP/1(r_SP1) -> r_SP1/1

== system detumbling_group24/Desturbances/External Torques/Solar radiation/Pressure ==
  Constant6 : Constant  Value=1358
  Constant7 : Constant  Value=c
  Product8 : Product
  Reciprocal : Product  Inputs=/
  P : Outport
  wires:
  Constant6/1 -> Product8/1
  Reciprocal/1 -> Product8/2
  Product8/1 -> P/1
  Constant7/1 -> Reciprocal/1

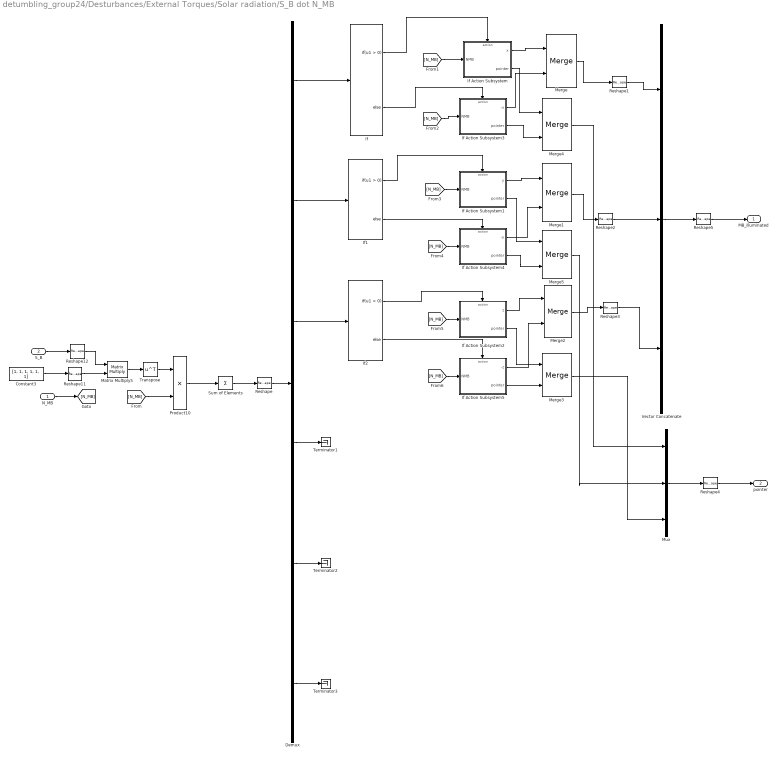
== system detumbling_group24/Desturbances/External Torques/Solar radiation/S_B dot N_MB ==
  N_MB : Inport
  S_B : Inport  Port=2
  Constant3 : Constant  Value=[1, 1, 1, 1, 1, 1]  VectorParams1D=off
  Demux : Demux  Outputs=6
  If : If
  If Action Subsystem : Subsystem  TreatAsAtomicUnit=on
  If Action Subsystem1 : Subsystem  TreatAsAtomicUnit=on
  If Action Subsystem2 : Subsystem  TreatAsAtomicUnit=on
  If Action Subsystem3 : Subsystem  TreatAsAtomicUnit=on
  If Action Subsystem4 : Subsystem  TreatAsAtomicUnit=on
  If Action Subsystem5 : Subsystem  TreatAsAtomicUnit=on
  If1 : If
  If2 : If
  Matrix Multiply5 : Product  Multiplication=Matrix(*)
  Merge{,1..5} (6 alike) : Merge
  Mux : Mux  Inputs=3
  Product10 : Product
  Reshape{,1..4,12} (6 alike) : Reshape  OutputDimensionality=Column vector (2-D)
  Reshape11 : Reshape  OutputDimensionality=Row vector (2-D)
  Reshape5 : Reshape  OutputDimensionality=Customize  OutputDimensions=[3,3]
  Sum of Elements : Sum  Inputs=+  CollapseMode=Specified dimension  CollapseDim=2
  Terminator1 : Terminator
  Terminator2 : Terminator
  Terminator3 : Terminator
  Transpose : Math  Operator=transpose
  Vector Concatenate : Concatenate  NumInputs=3
  MB_illuminated : Outport
  pointer : Outport  Port=2
  wires:
  Reshape12/1 -> Matrix Multiply5/1
  Matrix Multiply5/1 -> Transpose/1
  Product10/1 -> Sum of Elements/1
  Reshape11/1 -> Matrix Multiply5/2
  Constant3/1 -> Reshape11/1
  S_B/1 -> Reshape12/1
  Sum of Elements/1 -> Reshape/1
  Reshape/1 -> Demux/1
  Demux/1 -> If/1
  If/1 -> If Action Subsystem/Action
  If/2 -> If Action Subsystem3/Action
  N_MB/1 -> [N_MB]
  [N_MB] -> Product10/2
  [N_MB] -> If Action Subsystem/1(NMB)
  Demux/4 -> Terminator1/1
  Demux/5 -> Terminator2/1
  Demux/6 -> Terminator3/1
  Demux/2 -> If1/1
  If1/1 -> If Action Subsystem1/Action
  [N_MB] -> If Action Subsystem3/1(NMB)
  [N_MB] -> If Action Subsystem1/1(NMB)
  If1/2 -> If Action Subsystem4/Action
  [N_MB] -> If Action Subsystem4/1(NMB)
  If Action Subsystem3/1(-x) -> Merge/2
  If Action Subsystem/1(x) -> Merge/1
  If Action Subsystem1/1(y) -> Merge1/1
  If Action Subsystem2/1(z) -> Merge2/1
  If Action Subsystem5/1(-z) -> Merge2/2
  Demux/3 -> If2/1
  If2/1 -> If Action Subsystem2/Action
  If2/2 -> If Action Subsystem5/Action
  [N_MB] -> If Action Subsystem2/1(NMB)
  [N_MB] -> If Action Subsystem5/1(NMB)
  Merge/1 -> Reshape1/1
  Merge1/1 -> Reshape2/1
  Merge2/1 -> Reshape3/1
  Reshape1/1 -> Vector Concatenate/1
  Reshape2/1 -> Vector Concatenate/2
  Reshape3/1 -> Vector Concatenate/3
  Vector Concatenate/1 -> Reshape5/1
  If Action Subsystem4/1(-y) -> Merge1/2
  If Action Subsystem/2(pointer) -> Merge4/1
  If Action Subsystem3/2(pointer) -> Merge4/2
  If Action Subsystem1/2(pointer) -> Merge5/1
  If Action Subsystem4/2(pointer) -> Merge5/2
  If Action Subsystem2/2(pointer) -> Merge3/1
  If Action Subsystem5/2(pointer) -> Merge3/2
  Merge4/1 -> Mux/1
  Merge5/1 -> Mux/2
  Merge3/1 -> Mux/3
  Mux/1 -> Reshape4/1
  Reshape4/1 -> pointer/1
  Reshape5/1 -> MB_illuminated/1
  Transpose/1 -> Product10/1
